simulink model "kf_test"  (R2016b)
settings: Solver=VariableStepAuto  StartTime=0.0  StopTime=200.0  RelTol=1e-8
undefined symbols (not defined in the file): Continuous, Time
libraries: simulink x3, ctrlSharedLib x1
settings Model: Creator=Felles  LastModifiedBy=Felles

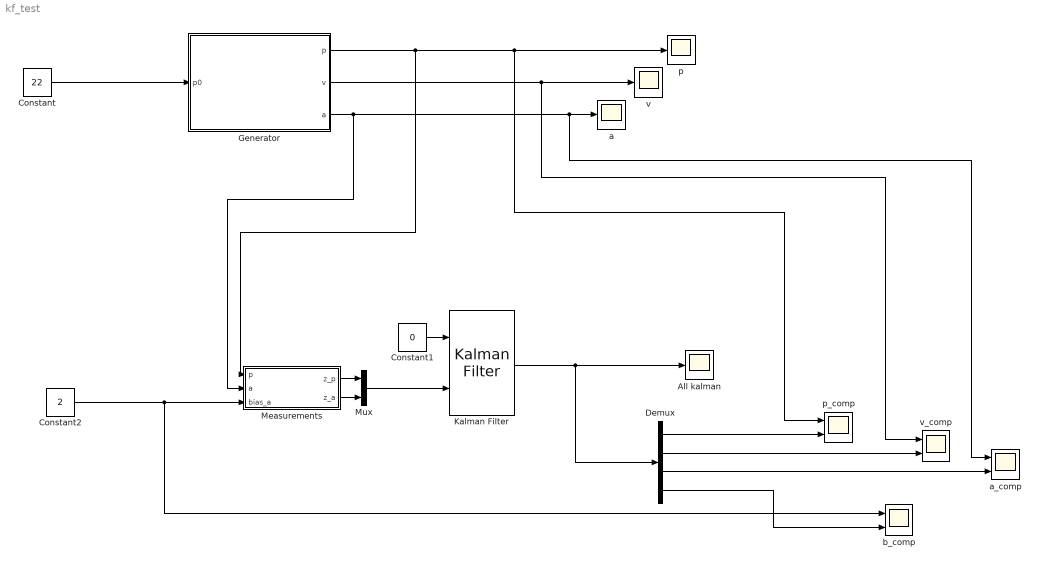
== system kf_test ==
  All kalman : Scope
  Constant : Constant  Value=22
  Constant1 : Constant  Value=0
  Constant2 : Constant  Value=2
  Demux : Demux
  Generator : Subsystem
  Kalman Filter : ctrlSharedLib/Kalman Filter  TimeDomain=Continuous-Time  UseCurrentEstimator=on  ModelSource=Individual A, B, C, D matrices  ModelSourceVariable=ss(0.95,1,1,0,1)  A=[0,1,0,0; 0,0,1,0; 0,0,0,0;0,0,0,0]  B=[0;0;0;0]  C=[1,0,0,0;0,0,1,1]  D=[0;0]  NumberOfStates=1  NumberOfInputs=1  NumberOfOutputs=1  InitialEstimateSource=Dialog  X0=[1 1 1 2.005]  P0=10  UseK=off  UseGH=off  NumberOfProcessNoiseInputs=1  G=1  TimeInvariantG=on  H=0  TimeInvariantH=on  Q=diag([1 1 1000 0.0001])  TimeInvariantQ=on  R=diag([1 1])  TimeInvariantR=on  N=0  TimeInvariantN=on  AddInputPort=on  AddEnablePort=off  ExternalReset=none  OutputEstimatedY=off  OutputP=off  Ts=-1
  Measurements : Subsystem
  Mux : Mux  Inputs=2
  a : Scope
  a_comp : Scope  NumInputPorts=2
  b_comp : Scope  NumInputPorts=2
  p : Scope
  p_comp : Scope  NumInputPorts=2
  v : Scope
  v_comp : Scope  NumInputPorts=2
  wires:
  Constant/1 -> Generator/1(p0)
  Generator/1(p) -> Measurements/1(p), p_comp/1, p/1
  Generator/2(v) -> v/1, v_comp/1
  Generator/3(a) -> Measurements/2(a), a_comp/1, a/1
  Constant1/1 -> Kalman Filter/1
  Mux/1 -> Kalman Filter/2
  Measurements/1(z_p) -> Mux/1
  Measurements/2(z_a) -> Mux/2
  Constant2/1 -> b_comp/1, Measurements/3(bias_a)
  Kalman Filter/1 -> Demux/1, All kalman/1
  Demux/2 -> v_comp/2
  Demux/1 -> p_comp/2
  Demux/3 -> a_comp/2
  Demux/4 -> b_comp/2

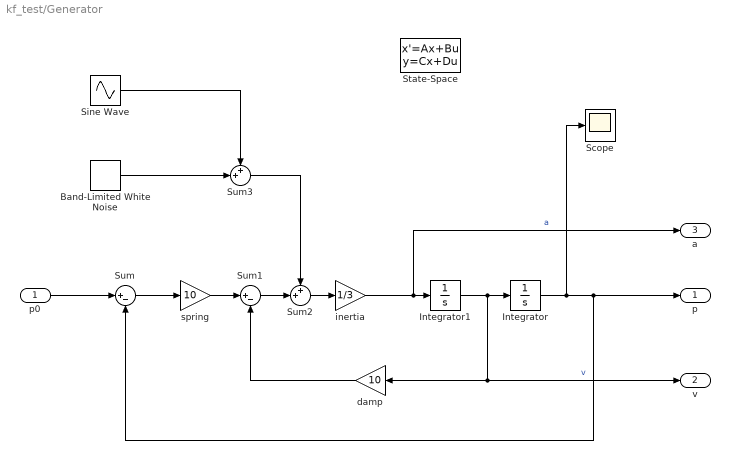
== system kf_test/Generator ==
  p0 : Inport
  Band-Limited White Noise : simulink/Sources/Band-Limited White Noise  Cov=[10]  Ts=0.1  seed=[23341]
  Integrator : Integrator
  Integrator1 : Integrator
  Scope : Scope
  Sine Wave : Sin  Amplitude=5  SampleTime=0
  State-Space : StateSpace  X0=0
  Sum : Sum  Inputs=|+-
  Sum1 : Sum  Inputs=|+-
  Sum2 : Sum  Inputs=++|
  Sum3 : Sum  Inputs=++|
  damp : Gain  Gain=10
  inertia : Gain  Gain=1/3
  spring : Gain  Gain=10
  p : Outport
  v : Outport  Port=2
  a : Outport  Port=3
  wires:
  p0/1 -> Sum/1
  Integrator1/1 -> damp/1, v/1, Integrator/1  "v"
  inertia/1 -> a/1, Integrator1/1  "a"
  Sum/1 -> spring/1
  Integrator/1 -> Scope/1, Sum/2, p/1
  damp/1 -> Sum1/2
  spring/1 -> Sum1/1
  Sum2/1 -> inertia/1
  Sum1/1 -> Sum2/2
  Band-Limited White Noise/1 -> Sum3/2
  Sine Wave/1 -> Sum3/1
  Sum3/1 -> Sum2/1

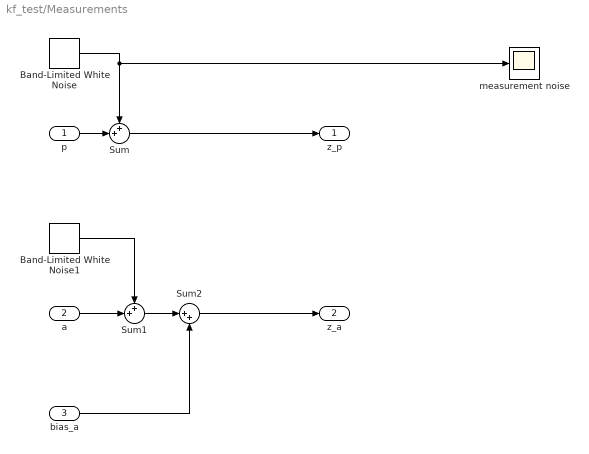
== system kf_test/Measurements ==
  p : Inport
  a : Inport  Port=2
  bias_a : Inport  Port=3
  Band-Limited White Noise : simulink/Sources/Band-Limited White Noise  Cov=[0.01]  Ts=0.1  seed=[23341]
  Band-Limited White Noise1 : simulink/Sources/Band-Limited White Noise  Cov=[0.01]  Ts=0.1  seed=[23341]
  Sum : Sum  Inputs=++|
  Sum1 : Sum  Inputs=++|
  Sum2 : Sum  Inputs=|++
  "measurement noise " : Scope
  z_p : Outport
  z_a : Outport  Port=2
  wires:
  p/1 -> Sum/2
  Sum/1 -> z_p/1
  Band-Limited White Noise/1 -> Sum/1, "measurement noise "/1
  a/1 -> Sum1/2
  Band-Limited White Noise1/1 -> Sum1/1
  Sum1/1 -> Sum2/1
  bias_a/1 -> Sum2/2
  Sum2/1 -> z_a/1
